simulink model "furuta_pen"  (R2017a)
settings: Solver=VariableStepAuto  StartTime=0.0  StopTime=10.0  RelTol=1e-3
values from neighbouring files (symbols this model uses):
  anpha_0 = 5    [ANN_params.m]    (also in furuta.m)
  beta0 = 5.8*10^(-4)    (= 0.00058)    [ANN_params.m]    (also in furuta.m)
  beta1 = 1.4142*10^(-3)    (= 0.0014142)    [ANN_params.m]    (also in furuta.m)
  g = 9.81    [ANN_params.m]    (also in furuta.m)
  J0 = 4.4*10^(-3)    (= 0.0044)    [ANN_params.m]    (also in furuta.m)
  J1 = 5.5026*10^(-4)    (= 0.00055026)    [ANN_params.m]    (also in furuta.m)
  ksw = 30    [furuta.m]
  L0 = 0.157    [ANN_params.m]    (also in furuta.m)
  L1 = 0.133    [ANN_params.m]    (also in furuta.m)
  m0 = 0.5355    [furuta.m]
  m1 = 0.078    [ANN_params.m]    (also in furuta.m = 0.0933)
  N = 1.05*eye(10)    [ANN_params.m]
  R = 8.53*eye(8)    [ANN_params.m]    (also in furuta.m = [-0.2500,20.6329,-0.6179,2.5406])
  theta_0 = 0    [ANN_params.m]    (also in furuta.m)
  up = 1    [furuta.m]
undefined symbols (not defined in the file or in its folder): X, Y, Z
libraries: sm_lib x12, nesl_utility x6
settings Model: Creator=Chechao  LastModifiedBy=chech
settings ExplorerConfigSet: InternalSimMechanicsExplorerSettings="<ExplorerConfiguration><canonicalview>planar_xy</canonicalview><AnimationSetting><BasePlaybackSpeed>1.0</BasePlaybackSpeed><PlaybackSpeedFactor>1.0</PlaybackSpeedFactor></AnimationSetting><TilePanel><TileInfo><Tiles Columns=\"1\" Count=\"1\" Rows=\"1\"><Column Left=\"2\" Weight=\"1\"/><Column Left=\"815\"/><Row Top=\"2\" Weight=\"1\"/><Row Top=\"278\"/><Tile Height=\"1\" Width=\"1\" X=\"0\" Y=\"0\"/></Tiles></TileInfo><SceneInfo><SceneViewer><BGColor><R>0.60000002384185791</R><G>0.60000002384185791</G><B>0.60000002384185791</B></BGColor><Camera><DoPerspective>off</DoPerspective><Position><X>3.0348189574883895</X><Y>0.89503316987109838</Y><Z>1.1148954709131602</Z></Position><Center><X>1.4216968578267744</X><Y>0.23812580067611089</Y><Z>-0.36954855728247171</Z></Center><Up><X>-0.074382553953715444</X><Y>0.93933115277276391</Y><Z>-0.3348495499443197</Z></Up><ViewLimDist>1</ViewLimDist><YLim>1.1431212443461942</YLim><XLim>3.4422077919638205</XLim></Camera></SceneViewer></SceneInfo></TilePanel><MechEditorPanel><Cameras/><GfxPanelCameraMap/><VideoCreator><PlaybackSpeedRatio>1.0</PlaybackSpeedRatio><FrameRate>30</FrameRate><VideoFormat>Motion JPEG AVI</VideoFormat><FrameSize>auto</FrameSize></VideoCreator></MechEditorPanel></ExplorerConfiguration>"

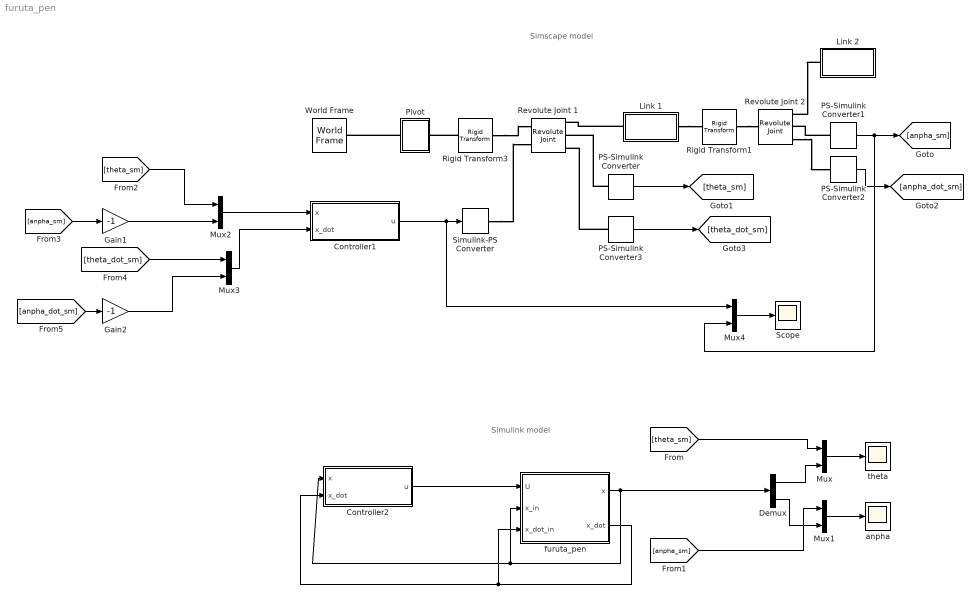
== system furuta_pen ==
  note: Simulink model
  note: Simscape model
  Controller1 : Subsystem
  Controller2 : Subsystem
  Demux : Demux  Outputs=2
  Gain1 : Gain  Gain=-1
  Gain2 : Gain  Gain=-1
  Link 1 : Subsystem  Tag=CustomStyle
  Link 2 : Subsystem  Tag=CustomStyle
  Mux{,1..4} (5 alike) : Mux  Inputs=2
  PS-Simulink Converter : nesl_utility/PS-Simulink Converter  PhysicalDomain=network_engine_domain  SubClassName=ps_output  LeftPortType=input  RightPortType=output  PseudoPeriodic=off  Frequencies=[]  Unit=rad  AffineConversion=off
  PS-Simulink Converter1 : nesl_utility/PS-Simulink Converter  PhysicalDomain=network_engine_domain  SubClassName=ps_output  LeftPortType=input  RightPortType=output  PseudoPeriodic=off  Frequencies=[]  Unit=rad  AffineConversion=off
  PS-Simulink Converter2 : nesl_utility/PS-Simulink Converter  PhysicalDomain=network_engine_domain  SubClassName=ps_output  LeftPortType=input  RightPortType=output  PseudoPeriodic=off  Frequencies=[]  Unit=rad/s  AffineConversion=off
  PS-Simulink Converter3 : nesl_utility/PS-Simulink Converter  PhysicalDomain=network_engine_domain  SubClassName=ps_output  LeftPortType=input  RightPortType=output  PseudoPeriodic=off  Frequencies=[]  Unit=rad/s  AffineConversion=off
  Pivot : Subsystem  Tag=CustomStyle
  Revolute Joint 1 : sm_lib/Joints/Revolute Joint  SenseConstraintForce=off  SenseConstraintForceX=off  SenseConstraintForceY=off  SenseConstraintForceZ=off  SenseConstraintTorque=off  SenseConstraintTorqueX=off  SenseConstraintTorqueY=off  SenseConstraintTorqueZ=off  SenseTotalForce=off  SenseTotalForceX=off  SenseTotalForceY=off  SenseTotalForceZ=off  SenseTotalTorque=off  SenseTotalTorqueX=off  SenseTotalTorqueY=off  SenseTotalTorqueZ=off  CompositeWrenchDir=FollowerOnBase  CompositeWrenchFrame=BaseFrame  EquilibriumPosition=0  EquilibriumPositionUnits=rad  SpringStiffness=0  SpringStiffnessUnits=N*m/rad  DampingCoefficient=beta0  DampingCoefficientUnits=N*m/(rad/s)  TorqueActuationMode=InputTorque  MotionActuationMode=ComputedMotion  SensePosition=on  SenseVelocity=on  SenseAcceleration=off  SenseTorqueForce=off  PositionTargetSpecify=on  PositionTargetPriority=High  PositionTargetValue=theta_0  PositionTargetValueUnits=deg  VelocityTargetSpecify=off  VelocityTargetPriority=High  VelocityTargetValue=0  VelocityTargetValueUnits=rad/s
  Revolute Joint 2 : sm_lib/Joints/Revolute Joint  SenseConstraintForce=off  SenseConstraintForceX=off  SenseConstraintForceY=off  SenseConstraintForceZ=off  SenseConstraintTorque=off  SenseConstraintTorqueX=off  SenseConstraintTorqueY=off  SenseConstraintTorqueZ=off  SenseTotalForce=off  SenseTotalForceX=off  SenseTotalForceY=off  SenseTotalForceZ=off  SenseTotalTorque=off  SenseTotalTorqueX=off  SenseTotalTorqueY=off  SenseTotalTorqueZ=off  CompositeWrenchDir=FollowerOnBase  CompositeWrenchFrame=BaseFrame  EquilibriumPosition=pi  EquilibriumPositionUnits=rad  SpringStiffness=0  SpringStiffnessUnits=N*m/rad  DampingCoefficient=beta1  DampingCoefficientUnits=N*m/(rad/s)  TorqueActuationMode=NoTorque  MotionActuationMode=ComputedMotion  SensePosition=on  SenseVelocity=on  SenseAcceleration=off  SenseTorqueForce=off  PositionTargetSpecify=on  PositionTargetPriority=High  PositionTargetValue=anpha_0  PositionTargetValueUnits=deg  VelocityTargetSpecify=off  VelocityTargetPriority=High  VelocityTargetValue=0  VelocityTargetValueUnits=rad/s
  Rigid Transform1 : sm_lib/Frames and Transforms/Rigid Transform  TranslationMethod=None  TranslationStandardOffset=0  TranslationLengthUnit=m  TranslationStandardAxis=+Z  TranslationCartesianOffset=[0 0 0]  TranslationROffset=0  TranslationROffsetUnits=m  TranslationZOffset=0  TranslationZOffsetUnits=m  TranslationThetaOffset=0  TranslationThetaOffsetUnits=deg  RotationMethod=StandardAxis  RotationAngleUnits=deg  RotationStandardAxis=-X  RotationAngle=90  RotationArbitraryAxis=[0 0 1]  FollAlignAxisA=+X  BaseAlignAxisA=+Y  FollAlignAxisB=+Y  BaseAlignAxisB=+Z  RotationSequenceAxes=FollowerAxes  RotationSequence=XYX  RotationSequenceAngles=[0 0 0]  RotationSequenceAnglesUnits=deg  RotationMatrix=[1 0 0; 0 1 0; 0 0 1]
  Rigid Transform3 : sm_lib/Frames and Transforms/Rigid Transform  TranslationMethod=StandardAxis  TranslationStandardOffset=0.25  TranslationLengthUnit=m  TranslationStandardAxis=+Z  TranslationCartesianOffset=[0 0 0]  TranslationROffset=0  TranslationROffsetUnits=m  TranslationZOffset=0  TranslationZOffsetUnits=m  TranslationThetaOffset=0  TranslationThetaOffsetUnits=deg  RotationMethod=None  RotationAngleUnits=deg  RotationStandardAxis=-X  RotationAngle=90  RotationArbitraryAxis=[0 0 1]  FollAlignAxisA=+X  BaseAlignAxisA=+Y  FollAlignAxisB=+Y  BaseAlignAxisB=+Z  RotationSequenceAxes=FollowerAxes  RotationSequence=XYX  RotationSequenceAngles=[0 0 0]  RotationSequenceAnglesUnits=deg  RotationMatrix=[1 0 0; 0 1 0; 0 0 1]
  Scope : Scope
  Simulink-PS Converter : nesl_utility/Simulink-PS Converter  PhysicalDomain=network_engine_domain  SubClassName=ps_input  LeftPortType=input  RightPortType=output  PseudoPeriodic=off  Frequencies=[]  NoiseDistribution=none  NoiseParameters=[]  Unit=1  AffineConversion=off  FilteringAndDerivatives=provide  SimscapeFilterOrder=1  InputFilterTimeConstant=0.001  UdotUserProvided=0
  World Frame : sm_lib/Frames and Transforms/World Frame
  anpha : Scope
  furuta_pen : Subsystem
  theta : Scope
  wires:
  furuta_pen/2(x_dot) -> Controller2/2(x_dot), furuta_pen/3(x_dot_in)
  furuta_pen/1(x) -> Demux/1, Controller2/1(x), furuta_pen/2(x_in)
  Controller2/1(u) -> furuta_pen/1(U)
  PS-Simulink Converter/1 -> [theta_sm]
  PS-Simulink Converter1/1 -> Mux4/2, [anpha_sm]
  Demux/1 -> Mux/2
  Mux/1 -> theta/1
  Mux1/1 -> anpha/1
  [theta_sm] -> Mux/1
  [anpha_sm] -> Mux1/1
  Demux/2 -> Mux1/2
  [theta_sm] -> Mux2/1
  [anpha_sm] -> Gain1/1
  Controller1/1(u) -> Mux4/1, Simulink-PS Converter/1
  PS-Simulink Converter2/1 -> [anpha_dot_sm]
  [theta_dot_sm] -> Mux3/1
  [anpha_dot_sm] -> Gain2/1
  Mux4/1 -> Scope/1
  Gain1/1 -> Mux2/2
  Gain2/1 -> Mux3/2
  Mux2/1 -> Controller1/1(x)
  Mux3/1 -> Controller1/2(x_dot)
  PS-Simulink Converter3/1 -> [theta_dot_sm]
  connections:
  Link 1/LConn1 -- Rigid Transform1/LConn1
  Link 1/RConn1 -- Revolute Joint 1/RConn1
  PS-Simulink Converter/LConn1 -- Revolute Joint 1/RConn2
  PS-Simulink Converter1/LConn1 -- Revolute Joint 2/RConn2
  Link 2/RConn1 -- Revolute Joint 2/RConn1
  Rigid Transform1/RConn1 -- Revolute Joint 2/LConn1
  Pivot/LConn1 -- World Frame/RConn1
  Rigid Transform3/LConn1 -- Pivot/RConn1
  Rigid Transform3/RConn1 -- Revolute Joint 1/LConn1
  Simulink-PS Converter/RConn1 -- Revolute Joint 1/LConn2
  Revolute Joint 2/RConn3 -- PS-Simulink Converter2/LConn1
  PS-Simulink Converter3/LConn1 -- Revolute Joint 1/RConn3

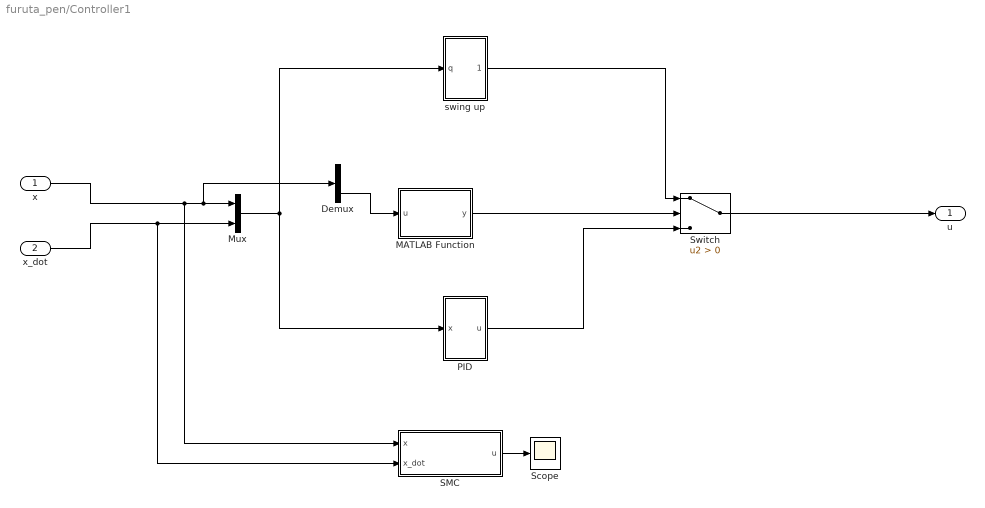
== system furuta_pen/Controller1 ==
  x : Inport
  x_dot : Inport  Port=2
  Demux : Demux  Outputs=2
  MATLAB Function : MATLAB Function  TreatAsAtomicUnit=on
  Mux : Mux  Inputs=2
  PID : Subsystem
  SMC : Subsystem
  Scope : Scope
  Switch : Switch  Criteria=u2 > Threshold
  swing up : Subsystem
  u : Outport
  wires:
  x/1 -> SMC/1(x), Demux/1, Mux/1
  x_dot/1 -> SMC/2(x_dot), Mux/2
  Mux/1 -> PID/1(x), swing up/1(q)
  Switch/1 -> u/1
  swing up/1(Out1) -> Switch/1
  MATLAB Function/1(y) -> Switch/2
  Demux/2 -> MATLAB Function/1(u)
  SMC/1(u) -> Scope/1
  PID/1(u) -> Switch/3

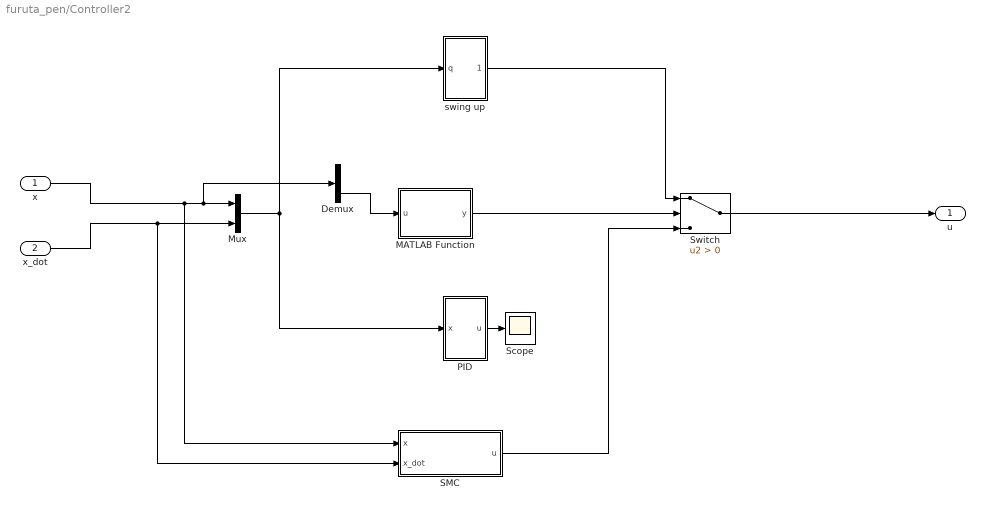
== system furuta_pen/Controller2 ==
  x : Inport
  x_dot : Inport  Port=2
  Demux : Demux  Outputs=2
  MATLAB Function : MATLAB Function  TreatAsAtomicUnit=on
  Mux : Mux  Inputs=2
  PID : Subsystem
  SMC : Subsystem
  Scope : Scope
  Switch : Switch  Criteria=u2 > Threshold
  swing up : Subsystem
  u : Outport
  wires:
  x/1 -> SMC/1(x), Demux/1, Mux/1
  x_dot/1 -> SMC/2(x_dot), Mux/2
  Mux/1 -> PID/1(x), swing up/1(q)
  Switch/1 -> u/1
  swing up/1(Out1) -> Switch/1
  MATLAB Function/1(y) -> Switch/2
  Demux/2 -> MATLAB Function/1(u)
  PID/1(u) -> Scope/1
  SMC/1(u) -> Switch/3

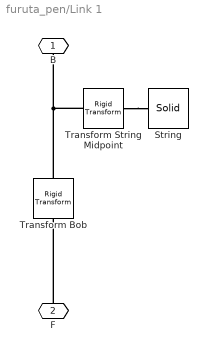
== system furuta_pen/Link 1 ==
  String : sm_lib/Body Elements/Solid  InertiaType=CalculateFromGeometry  Mass=m0  MassUnits=kg  CenterOfMass=[0 0 0]  CenterOfMassUnits=m  MomentsOfInertia=[1 1 1]*1e-3  MomentsOfInertiaUnits=kg*m^2  ProductsOfInertia=[0 0 0]  ProductsOfInertiaUnits=kg*m^2  DensityBased=off  Density=2700  DensityUnits=kg/(m^3)  DoExposeReferenceFrame=on  SerializedFrames=<Frames/>  GraphicType=FromGeometry  MarkerShape=Sphere  MarkerSize=10  MarkerSizeUnits=m  GraphicVisPropType=SimpleVisualProperties  GraphicDiffuseColor=[1.0 0.2 0.0]  GraphicSpecularColor=[0.5 0.5 0.5 1.0]  GraphicAmbientColor=[0.15 0.15 0.15 1.0]  GraphicEmissiveColor=[0.0 0.0 0.0 1.0]  GraphicShininess=75  GraphicOpacity=1.0  GeometryShape=Brick  RectangleSize=[1 1]  RectangleSizeUnits=m  BrickDimensions=[0.01 L0 0.01]  BrickDimensionUnits=m  CylinderRadius=0.1  CylinderRadiusUnits=m  CylinderLength=1  CylinderLengthUnits=m  SphereRadius=0.1  SphereRadiusUnits=m  EllipsoidRadii=[1 1 1]  EllipsoidRadiiUnits=m  ExtrusionCrossSection=[1 1; -1 1; -1 -1; 1 -1]  ExtrusionCrossSectionUnits=m  ExtrusionLength=1  ExtrusionLengthUnits=m  PolygonNumSides=3  PolygonOuterRadius=1  PolygonOuterRadiusUnits=m  ExtGeomFileType=STL  ExtGeomFileUnits=m  RevolutionCrossSection=[1 1; 1 -1; 2 -1; 2 1]  RevolutionCrossSectionUnits=m  RevolutionExtent=Full  RevolutionAngle=180  RevolutionAngleUnits=deg
  "Transform Bob " : sm_lib/Frames and Transforms/Rigid Transform  TranslationMethod=StandardAxis  TranslationStandardOffset=L0  TranslationLengthUnit=m  TranslationStandardAxis=-Y  TranslationCartesianOffset=[0 0 0]  TranslationROffset=0  TranslationROffsetUnits=m  TranslationZOffset=0  TranslationZOffsetUnits=m  TranslationThetaOffset=0  TranslationThetaOffsetUnits=deg  RotationMethod=None  RotationAngleUnits=deg  RotationStandardAxis=+Z  RotationAngle=0  RotationArbitraryAxis=[0 0 1]  FollAlignAxisA=+X  BaseAlignAxisA=+Y  FollAlignAxisB=+Y  BaseAlignAxisB=+Z  RotationSequenceAxes=FollowerAxes  RotationSequence=XYX  RotationSequenceAngles=[0 0 0]  RotationSequenceAnglesUnits=deg  RotationMatrix=[1 0 0; 0 1 0; 0 0 1]
  Transform String Midpoint : sm_lib/Frames and Transforms/Rigid Transform  TranslationMethod=StandardAxis  TranslationStandardOffset=L0/2  TranslationLengthUnit=m  TranslationStandardAxis=-Y  TranslationCartesianOffset=[0 0 0]  TranslationROffset=0  TranslationROffsetUnits=m  TranslationZOffset=0  TranslationZOffsetUnits=m  TranslationThetaOffset=0  TranslationThetaOffsetUnits=deg  RotationMethod=None  RotationAngleUnits=deg  RotationStandardAxis=+Z  RotationAngle=0  RotationArbitraryAxis=[0 0 1]  FollAlignAxisA=+X  BaseAlignAxisA=+Y  FollAlignAxisB=+Y  BaseAlignAxisB=+Z  RotationSequenceAxes=FollowerAxes  RotationSequence=XYX  RotationSequenceAngles=[0 0 0]  RotationSequenceAnglesUnits=deg  RotationMatrix=[1 0 0; 0 1 0; 0 0 1]
  B : PMIOPort  Port=1  Side=Right
  F : PMIOPort  Port=2  Side=Left
  connections:
  "Transform Bob "/LConn1 -- Transform String Midpoint/LConn1 -- B/RConn1
  F/RConn1 -- "Transform Bob "/RConn1
  Transform String Midpoint/RConn1 -- String/RConn1

== system furuta_pen/Link 2 ==
  String : sm_lib/Body Elements/Solid  InertiaType=CalculateFromGeometry  Mass=m1  MassUnits=kg  CenterOfMass=[0 0 0]  CenterOfMassUnits=m  MomentsOfInertia=[1 1 1]*1e-3  MomentsOfInertiaUnits=kg*m^2  ProductsOfInertia=[0 0 0]  ProductsOfInertiaUnits=kg*m^2  DensityBased=off  Density=2700  DensityUnits=kg/(m^3)  DoExposeReferenceFrame=on  SerializedFrames=<Frames/>  GraphicType=FromGeometry  MarkerShape=Sphere  MarkerSize=10  MarkerSizeUnits=m  GraphicVisPropType=SimpleVisualProperties  GraphicDiffuseColor=[0.2 1.0 0.8]  GraphicSpecularColor=[0.5 0.5 0.5 1.0]  GraphicAmbientColor=[0.15 0.15 0.15 1.0]  GraphicEmissiveColor=[0.0 0.0 0.0 1.0]  GraphicShininess=75  GraphicOpacity=1.0  GeometryShape=Brick  RectangleSize=[1 1]  RectangleSizeUnits=m  BrickDimensions=[0.01 2*L1 0.01]  BrickDimensionUnits=m  CylinderRadius=0.1  CylinderRadiusUnits=m  CylinderLength=1  CylinderLengthUnits=m  SphereRadius=0.1  SphereRadiusUnits=m  EllipsoidRadii=[1 1 1]  EllipsoidRadiiUnits=m  ExtrusionCrossSection=[1 1; -1 1; -1 -1; 1 -1]  ExtrusionCrossSectionUnits=m  ExtrusionLength=1  ExtrusionLengthUnits=m  PolygonNumSides=3  PolygonOuterRadius=1  PolygonOuterRadiusUnits=m  ExtGeomFileType=STL  ExtGeomFileUnits=m  RevolutionCrossSection=[1 1; 1 -1; 2 -1; 2 1]  RevolutionCrossSectionUnits=m  RevolutionExtent=Full  RevolutionAngle=180  RevolutionAngleUnits=deg
  Transform String Midpoint : sm_lib/Frames and Transforms/Rigid Transform  TranslationMethod=StandardAxis  TranslationStandardOffset=L1  TranslationLengthUnit=m  TranslationStandardAxis=-Y  TranslationCartesianOffset=[0 0 0]  TranslationROffset=0  TranslationROffsetUnits=m  TranslationZOffset=0  TranslationZOffsetUnits=m  TranslationThetaOffset=0  TranslationThetaOffsetUnits=deg  RotationMethod=None  RotationAngleUnits=deg  RotationStandardAxis=+Z  RotationAngle=0  RotationArbitraryAxis=[0 0 1]  FollAlignAxisA=+X  BaseAlignAxisA=+Y  FollAlignAxisB=+Y  BaseAlignAxisB=+Z  RotationSequenceAxes=FollowerAxes  RotationSequence=XYX  RotationSequenceAngles=[0 0 0]  RotationSequenceAnglesUnits=deg  RotationMatrix=[1 0 0; 0 1 0; 0 0 1]
  B : PMIOPort  Port=1  Side=Right
  connections:
  Transform String Midpoint/RConn1 -- String/RConn1
  Transform String Midpoint/LConn1 -- B/RConn1

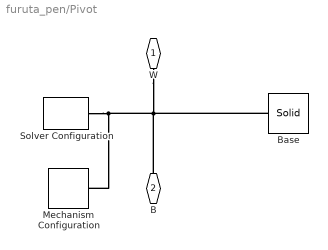
== system furuta_pen/Pivot ==
  Base : sm_lib/Body Elements/Solid  InertiaType=CalculateFromGeometry  Mass=1  MassUnits=kg  CenterOfMass=[0 0 0]  CenterOfMassUnits=m  MomentsOfInertia=[1 1 1]*1e-3  MomentsOfInertiaUnits=kg*m^2  ProductsOfInertia=[0 0 0]  ProductsOfInertiaUnits=kg*m^2  DensityBased=on  Density=1000  DensityUnits=kg/(m^3)  DoExposeReferenceFrame=on  SerializedFrames=<Frames/>  GraphicType=FromGeometry  MarkerShape=Sphere  MarkerSize=10  MarkerSizeUnits=m  GraphicVisPropType=SimpleVisualProperties  GraphicDiffuseColor=[0.2 0.2 0.2]  GraphicSpecularColor=[0.5 0.5 0.5 1.0]  GraphicAmbientColor=[0.15 0.15 0.15 1.0]  GraphicEmissiveColor=[0.0 0.0 0.0 1.0]  GraphicShininess=75  GraphicOpacity=1.0  GeometryShape=Cylinder  RectangleSize=[1 1]  RectangleSizeUnits=m  BrickDimensions=[1 0.1 0.1]  BrickDimensionUnits=m  CylinderRadius=0.1  CylinderRadiusUnits=m  CylinderLength=0.5  CylinderLengthUnits=m  SphereRadius=0.1  SphereRadiusUnits=m  EllipsoidRadii=[1 1 1]  EllipsoidRadiiUnits=m  ExtrusionCrossSection=[1 1; -1 1; -1 -1; 1 -1]  ExtrusionCrossSectionUnits=m  ExtrusionLength=1  ExtrusionLengthUnits=m  PolygonNumSides=3  PolygonOuterRadius=1  PolygonOuterRadiusUnits=m  ExtGeomFileType=STL  ExtGeomFileUnits=m  RevolutionCrossSection=[1 1; 1 -1; 2 -1; 2 1]  RevolutionCrossSectionUnits=m  RevolutionExtent=Full  RevolutionAngle=180  RevolutionAngleUnits=deg
  Mechanism Configuration : sm_lib/Utilities/Mechanism Configuration  UniformGravity=Constant  GravityVector=[0 0 -g]  GravityUnits=m/s^2  LinearizationDelta=0.001
  Solver Configuration : nesl_utility/Solver Configuration  PhysicalDomain=network_engine_domain  SubClassName=solver  LeftPortType=input  RightPortType=generic  Accelerate=off  Tones=[]  Harmonics=[]  SimulateNoise=off  Profile=off  UseLocalSampling=off  EnableSwitchedLinearOptims=on  FrequencyDomain=off  UseCCode=off  RelTol=0.001  AbsTol=1e-06  MinStep=1e-09  ToWorkspace=off  RevertToSquareIcSolve=off  NumHomotopyIterations=100  PhasorMode=off  PhasorModeNumHarmonics=1  OverrideAbsTol=off  DoDC=off  ResidualTolerance=1e-9  UseLocalSolver=off  LocalSolverChoice=NE_BACKWARD_EULER_ADVANCER  LocalSolverSampleTime=.001  DoFixedCost=off  MaxNonlinIter=3  MaxModeIter=2  LinearAlgebra=Sparse  DelaysMemoryBudget=1024  AutomaticFiltering=on  FilteringTimeConstant=0.001
  W : PMIOPort  Port=1  Side=Left
  B : PMIOPort  Port=2  Side=Right
  connections:
  W/RConn1 -- B/RConn1 -- Base/RConn1 -- Solver Configuration/RConn1 -- Mechanism Configuration/RConn1

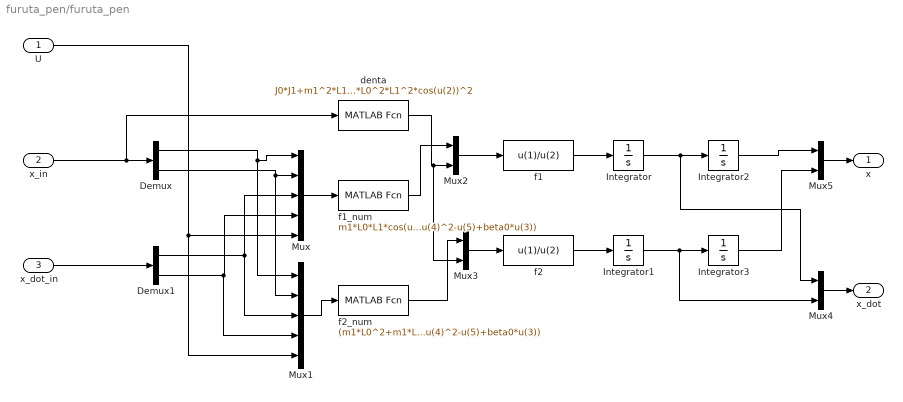
== system furuta_pen/furuta_pen ==
  U : Inport
  x_in : Inport  Port=2
  x_dot_in : Inport  Port=3
  Demux : Demux  Outputs=2
  Demux1 : Demux  Outputs=2
  Integrator : Integrator
  Integrator1 : Integrator
  Integrator2 : Integrator  InitialCondition=theta_0*pi/180
  Integrator3 : Integrator  InitialCondition=anpha_0/180*pi
  Mux : Mux  Inputs=5
  Mux1 : Mux  Inputs=5
  Mux{2..5} (4 alike) : Mux  Inputs=2
  denta : MATLABFcn  MATLABFcn=J0*J1+m1^2*L1^4*sin(u(2))^2+m1^2*L0^2*L1^2+J0*m1*L1^2+J1*m1*L0^2+J1*m1*L1^2*sin(u(2))^2-m1^2*L0^2*L1^2*cos(u(2))^2
  f1 : MATLABFcn  MATLABFcn=u(1)/u(2)
  f1_num : MATLABFcn  MATLABFcn=m1*L0*L1*cos(u(2))*(0.5*m1*L1^2*sin(2*u(2))*u(3)^2+m1*g*L1*sin(u(2))-beta1*u(4))-(m1*L1^2+J1)*(m1*L1^2*sin(2*u(2))*u(3)*u(4)+m1*L0*L1*sin(u(2))*u(4)^2-u(5)+beta0*u(3))
  f2 : MATLABFcn  MATLABFcn=u(1)/u(2)
  f2_num : MATLABFcn  MATLABFcn=(m1*L0^2+m1*L1^2*sin(u(2))^2+J0)*(0.5*m1*L1^2*sin(2*u(2))*u(3)^2+m1*g*L1*sin(u(2))-beta1*u(4))-m1*L0*L1*cos(u(2))*(m1*L1^2*sin(2*u(2))*u(3)*u(4)+m1*L0*L1*sin(u(2))*u(4)^2-u(5)+beta0*u(3))
  x : Outport
  x_dot : Outport  Port=2
  wires:
  x_in/1 -> Demux/1, denta/1
  Mux/1 -> f1_num/1
  Mux1/1 -> f2_num/1
  Mux2/1 -> f1/1
  denta/1 -> Mux3/2, Mux2/2
  f1_num/1 -> Mux2/1
  Mux3/1 -> f2/1
  f2_num/1 -> Mux3/1
  f1/1 -> Integrator/1
  f2/1 -> Integrator1/1
  Integrator/1 -> Mux4/1, Integrator2/1
  Integrator1/1 -> Mux4/2, Integrator3/1
  Mux4/1 -> x_dot/1
  Mux5/1 -> x/1
  Integrator2/1 -> Mux5/1
  Integrator3/1 -> Mux5/2
  U/1 -> Mux1/5, Mux/5
  x_dot_in/1 -> Demux1/1
  Demux/1 -> Mux1/1, Mux/1
  Demux/2 -> Mux1/2, Mux/2
  Demux1/2 -> Mux1/4, Mux/4
  Demux1/1 -> Mux1/3, Mux/3

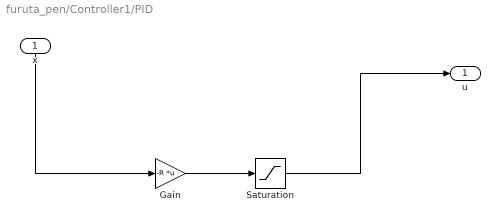
== system furuta_pen/Controller1/PID ==
  x : Inport
  Gain : Gain  Gain=-R  Multiplication=Matrix(K*u)
  Saturation : Saturate  UpperLimit=up  LowerLimit=-up
  u : Outport
  wires:
  Saturation/1 -> u/1
  x/1 -> Gain/1
  Gain/1 -> Saturation/1

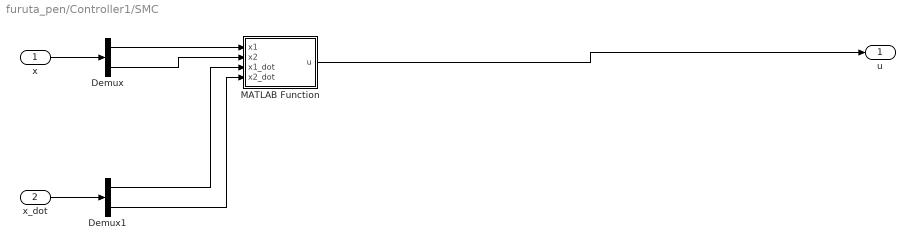
== system furuta_pen/Controller1/SMC ==
  x : Inport
  x_dot : Inport  Port=2
  Demux : Demux  Outputs=2
  Demux1 : Demux  Outputs=2
  MATLAB Function : MATLAB Function  TreatAsAtomicUnit=on
  u : Outport
  wires:
  MATLAB Function/1(u) -> u/1
  x/1 -> Demux/1
  Demux/1 -> MATLAB Function/1(x1)
  Demux/2 -> MATLAB Function/2(x2)
  Demux1/1 -> MATLAB Function/3(x1_dot)
  Demux1/2 -> MATLAB Function/4(x2_dot)
  x_dot/1 -> Demux1/1

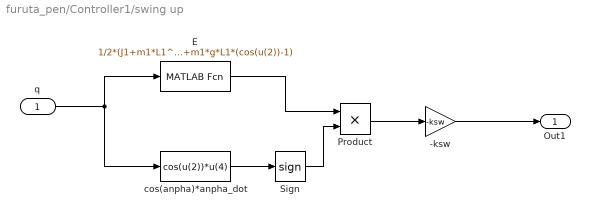
== system furuta_pen/Controller1/swing up ==
  q : Inport
  -ksw : Gain  Gain=-ksw
  E : MATLABFcn  MATLABFcn=1/2*(J1+m1*L1^2)*u(4)^2+m1*g*L1*(cos(u(2))-1)
  Product : Product
  Sign : Signum
  cos(anpha)*anpha_dot : MATLABFcn  MATLABFcn=cos(u(2))*u(4)
  Out1 : Outport
  wires:
  Sign/1 -> Product/2
  E/1 -> Product/1
  Product/1 -> -ksw/1
  cos(anpha)*anpha_dot/1 -> Sign/1
  q/1 -> E/1, cos(anpha)*anpha_dot/1
  -ksw/1 -> Out1/1

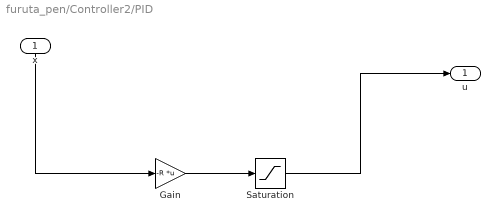
== system furuta_pen/Controller2/PID ==
  x : Inport
  Gain : Gain  Gain=-R  Multiplication=Matrix(K*u)
  Saturation : Saturate  UpperLimit=up  LowerLimit=-up
  u : Outport
  wires:
  Saturation/1 -> u/1
  x/1 -> Gain/1
  Gain/1 -> Saturation/1

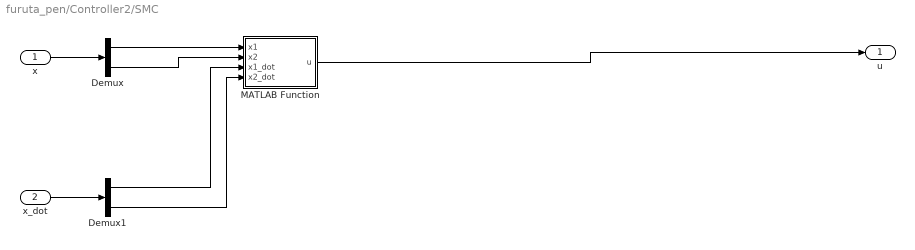
== system furuta_pen/Controller2/SMC ==
  x : Inport
  x_dot : Inport  Port=2
  Demux : Demux  Outputs=2
  Demux1 : Demux  Outputs=2
  MATLAB Function : MATLAB Function  TreatAsAtomicUnit=on
  u : Outport
  wires:
  MATLAB Function/1(u) -> u/1
  x/1 -> Demux/1
  Demux/1 -> MATLAB Function/1(x1)
  Demux/2 -> MATLAB Function/2(x2)
  Demux1/1 -> MATLAB Function/3(x1_dot)
  Demux1/2 -> MATLAB Function/4(x2_dot)
  x_dot/1 -> Demux1/1

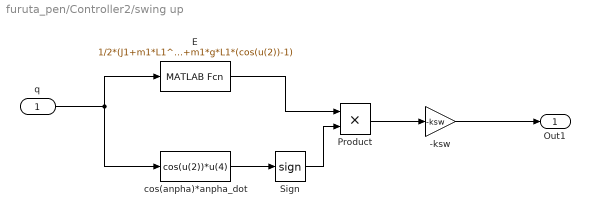
== system furuta_pen/Controller2/swing up ==
  q : Inport
  -ksw : Gain  Gain=-ksw
  E : MATLABFcn  MATLABFcn=1/2*(J1+m1*L1^2)*u(4)^2+m1*g*L1*(cos(u(2))-1)
  Product : Product
  Sign : Signum
  cos(anpha)*anpha_dot : MATLABFcn  MATLABFcn=cos(u(2))*u(4)
  Out1 : Outport
  wires:
  Sign/1 -> Product/2
  E/1 -> Product/1
  Product/1 -> -ksw/1
  cos(anpha)*anpha_dot/1 -> Sign/1
  q/1 -> E/1, cos(anpha)*anpha_dot/1
  -ksw/1 -> Out1/1

== matlab function furuta_pen/Controller2/MATLAB Function ==
  data: u input; y output
function y = fcn(u)
if abs(u)<20*pi/180
    y = 0;
else
    y= 1;
end

== matlab function furuta_pen/Controller1/SMC/MATLAB Function ==
  data: x1 input; u output; x2 input; x1_dot input; x2_dot input
function u = fcn(x1,x2,x1_dot,x2_dot)
b = [14.8452;12.5278];
C = [0,17.3564;
    0,67.377];
D = [-0.1172,-0.2411;
    -0.0989,-0.09359];
M = [0.5,0;
    0,10];
Q= [5/16,-3/4;
    -3/4,9/4];
R = [161/160 -3;
    -3 9];
x = [x1;x2];
x_dot = [x1_dot;x2_dot];
s = M*x+x_dot;
u = -(s'*R*s+s'*Q*(M+D)*x_dot+s'*Q*C*x)/(s'*Q*b);

== matlab function furuta_pen/Controller2/SMC/MATLAB Function ==
  data: x1 input; u output; x2 input; x1_dot input; x2_dot input
function u = fcn(x1,x2,x1_dot,x2_dot)
b = [14.8452;12.5278];
C = [0,17.3564;
    0,67.377];
D = [-0.1172,-0.2411;
    -0.0989,-0.09359];
M = [0.5,0;
    0,10];
Q= [5/16,-3/4;
    -3/4,9/4];
R = [161/160 -3;
    -3 9];
x = [x1;x2];
x_dot = [x1_dot;x2_dot];
s = M*x+x_dot;
u = -(s'*R*s+s'*Q*(M+D)*x_dot+s'*Q*C*x)/(s'*Q*b);

== matlab function furuta_pen/Controller1/MATLAB Function ==
  data: u input; y output
function y = fcn(u)
if abs(u)<20*pi/180
    y = 0;
else
    y= 1;
end
